simulink subsystem "PieroCPZ"  (R2023b)
settings: Solver=VariableStepAuto  StartTime=0.0  StopTime=10.0  RelTol=1e-3
settings Model: Creator=Carlos  LastModifiedBy=Carlos

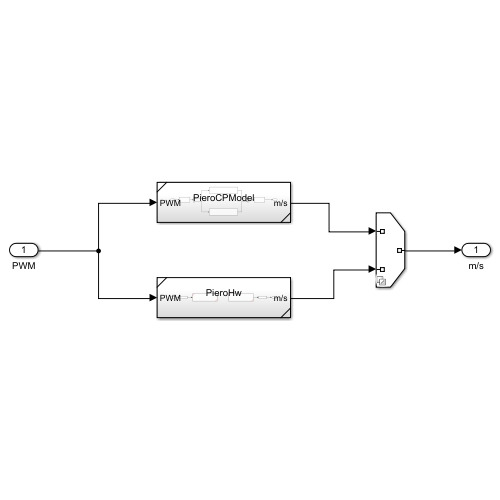
[thumbnail: Simulink's stored preview of the top-level diagram]
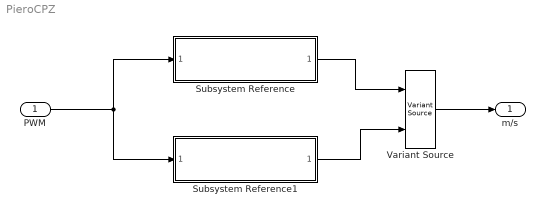
== system PieroCPZ ==
  PWM : Inport
  Subsystem Reference : Subsystem  ReferencedSubsystem=PieroCPModelZ
  Subsystem Reference1 : Subsystem  ReferencedSubsystem=PieroHwZ
  Variant Source : VariantSource  VariantControlMode=sim codegen switching
  m/s : Outport
  wires:
  PWM/1 -> Subsystem Reference/1, Subsystem Reference1/1
  Variant Source/1 -> m/s/1
  Subsystem Reference/1 -> Variant Source/1
  Subsystem Reference1/1 -> Variant Source/2
